simulink model "pendulo_pv"  (R2020b)
settings: Solver=FixedStepAuto  StartTime=0.0  StopTime=100  FixedStep=1e-3  RelTol=1e-3
values from neighbouring files (symbols this model uses):
  controlador = projetarControlador(requisitos, planta)    [executarTudo.m]    (also in runAll.m = projetarControladorPV(requisitos, planta))
  planta = obterPlanta()    [codetest.m]    (also in executarTudo.m; nextState.m; runAll.m)
  thetar = 0    [executarTudo.m]    (also in runAll.m)
  varCom = 0.01    [runAll.m]
  varMed = 0.001    [runAll.m]
settings Model: Creator=davi  LastModifiedBy=alexandremaranhao

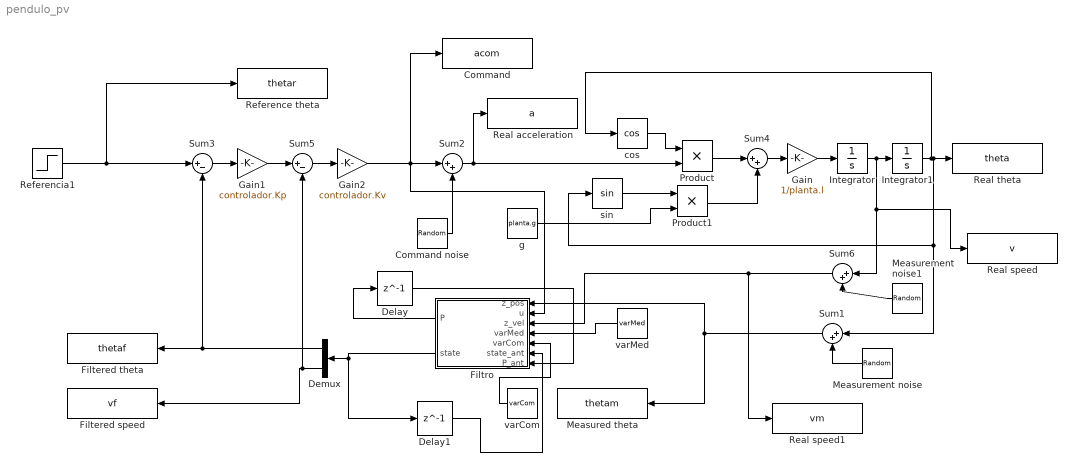
== system pendulo_pv ==
  Command : ToWorkspace  VariableName=acom  SaveFormat=Structure With Time  SampleTime=-1
  Command noise : RandomNumber  Variance=varCom  SampleTime=1e-2
  Delay : Delay  DelayLength=1  InitialCondition=eye(2)  SampleTime=1e-2
  Delay1 : Delay  DelayLength=1  InitialCondition=[0;0]  SampleTime=1e-2
  Demux : Demux  Outputs=2
  Filtered speed : ToWorkspace  VariableName=vf  SaveFormat=Structure With Time  SampleTime=-1
  Filtered theta : ToWorkspace  VariableName=thetaf  SaveFormat=Structure With Time  SampleTime=-1
  Filtro : MATLAB Function  TreatAsAtomicUnit=on  SystemSampleTime=1e-2
  Gain : Gain  Gain=1/planta.l
  Gain1 : Gain  Gain=controlador.Kp
  Gain2 : Gain  Gain=controlador.Kv
  Integrator : Integrator
  Integrator1 : Integrator
  Measured theta : ToWorkspace  VariableName=thetam  SaveFormat=Structure With Time  SampleTime=-1
  Measurement noise : RandomNumber  Variance=varMed  SampleTime=1e-2
  Measurement noise1 : RandomNumber  Variance=varMed  SampleTime=1e-2
  Product : Product
  Product1 : Product
  Real acceleration : ToWorkspace  VariableName=a  SaveFormat=Structure With Time  SampleTime=-1
  Real speed : ToWorkspace  VariableName=v  SaveFormat=Structure With Time  SampleTime=-1
  Real speed1 : ToWorkspace  VariableName=vm  SaveFormat=Structure With Time  SampleTime=-1
  Real theta : ToWorkspace  VariableName=theta  SaveFormat=Structure With Time  SampleTime=-1
  Reference theta : ToWorkspace  VariableName=thetar  SaveFormat=Structure With Time  SampleTime=-1
  Referencia1 : Step  Time=0  After=thetar  SampleTime=0
  Sum{1..2,4,6} (4 alike) : Sum  Inputs=|++
  Sum3 : Sum  Inputs=|+-
  Sum5 : Sum  Inputs=|+-
  cos : Trigonometry  Operator=cos
  g : Constant  Value=planta.g
  sin : Trigonometry
  varCom : Constant  Value=varCom
  varMed : Constant  Value=varMed
  wires:
  Product/1 -> Sum4/1
  Measurement noise/1 -> Sum1/2
  Sum2/1 -> Product/2, Real acceleration/1
  Command noise/1 -> Sum2/2
  Referencia1/1 -> Sum3/1, Reference theta/1
  cos/1 -> Product/1
  sin/1 -> Product1/1
  g/1 -> Product1/2
  Product1/1 -> Sum4/2
  Sum4/1 -> Gain/1
  Gain/1 -> Integrator/1
  Integrator/1 -> Sum6/1, Real speed/1, Integrator1/1
  Integrator1/1 -> sin/1, Sum1/1, Real theta/1, cos/1
  Sum3/1 -> Gain1/1
  varMed/1 -> Filtro/4(varMed)
  varCom/1 -> Filtro/5(varCom)
  Sum1/1 -> Measured theta/1, Filtro/1(z_pos)
  Filtro/2(state) -> Delay1/1, Demux/1
  Filtro/1(P) -> Delay/1
  Delay1/1 -> Filtro/6(state_ant)
  Delay/1 -> Filtro/7(P_ant)
  Demux/2 -> Filtered speed/1, Sum5/2
  Demux/1 -> Sum3/2, Filtered theta/1
  Gain2/1 -> Filtro/2(u), Command/1, Sum2/1
  Gain1/1 -> Sum5/1
  Sum5/1 -> Gain2/1
  Measurement noise1/1 -> Sum6/2
  Sum6/1 -> Real speed1/1, Filtro/3(z_vel)

== matlab function pendulo_pv/Filtro ==
  settings: updateMethod=DISCRETE
  data: z_pos input; u input; z_vel input; varMed input; varCom input; state_ant input; P_ant input; P output; state output
function [P, state] = fcn(z_pos, u, z_vel, varMed, varCom, state_ant, P_ant)

F = [1.0010    0.0100; 0.1963    1.0010];
G = [0.0001; 0.02];
n=2;
Q=G*varCom*G'; %covariance of process
R=varMed*eye(2);        %covariance of measurement  

x_pred = F*state_ant + G*u;
P_pred = F*P_ant*F' + Q;

C = [1 0;0 1];
z = [z_pos; z_vel];
Kt = P_pred * C' * pinv(R + C*P_pred*C');
state = x_pred + Kt*(z-C*state_ant);
P = P_pred - Kt*C*P_pred;
% y = z;
end
